simulink model "direct_2"  (Simulink 7.6)
settings: Solver=ode45  StartTime=0.0  StopTime=10.0  RelTol=1e-3
libraries: simulink x3
settings Model: Creator=Docencia  LastModifiedBy=Docencia

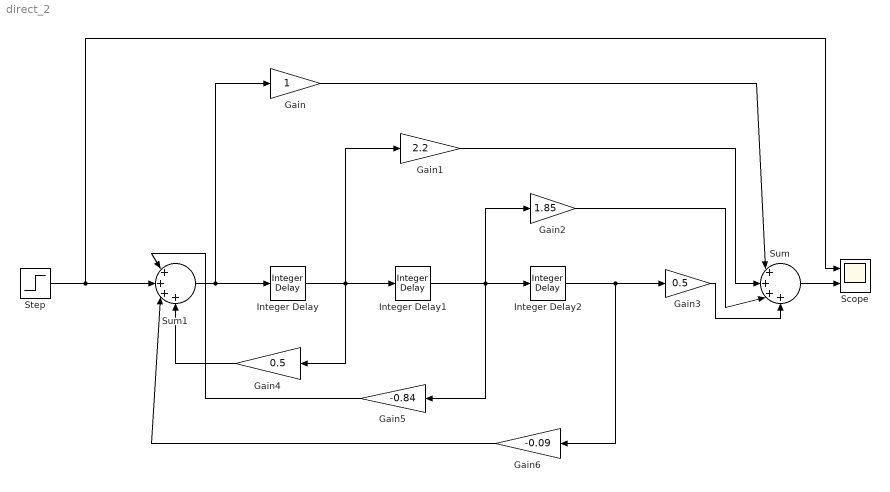
== system direct_2 ==
  Gain : Gain
  Gain1 : Gain  Gain=2.2
  Gain2 : Gain  Gain=1.85
  Gain3 : Gain  Gain=0.5
  Gain4 : Gain  Gain=0.5
  Gain5 : Gain  Gain=-0.84
  Gain6 : Gain  Gain=-0.09
  Integer Delay : simulink/Discrete/Integer Delay  NumDelays=1  vinit=0.0  samptime=-1
  Integer Delay1 : simulink/Discrete/Integer Delay  NumDelays=1  vinit=0.0  samptime=-1
  Integer Delay2 : simulink/Discrete/Integer Delay  NumDelays=1  vinit=0.0  samptime=-1
  Scope : Scope  NumInputPorts=2
      settings: YMin=-5~-5  YMax=5~5
  Step : Step  Time=2  SampleTime=0
  Sum : Sum  Inputs=|++++
  Sum1 : Sum  Inputs=|++++
  wires:
  Step/1 -> Scope/1, Sum1/2
  Integer Delay/1 -> Integer Delay1/1, Gain1/1, Gain4/1
  Integer Delay1/1 -> Integer Delay2/1, Gain2/1, Gain5/1
  Integer Delay2/1 -> Gain3/1, Gain6/1
  Gain/1 -> Sum/1
  Gain1/1 -> Sum/2
  Gain2/1 -> Sum/3
  Gain3/1 -> Sum/4
  Sum1/1 -> Integer Delay/1, Gain/1
  Gain6/1 -> Sum1/3
  Gain5/1 -> Sum1/1
  Sum/1 -> Scope/2
  Gain4/1 -> Sum1/4
